simulink model "enabled_triggered_ejemplo"  (Simulink 7.1)
settings: Solver=ode45  StartTime=0.0  StopTime=10.0  RelTol=1e-3
settings Model: Creator=Usuario  LastModifiedBy=Usuario

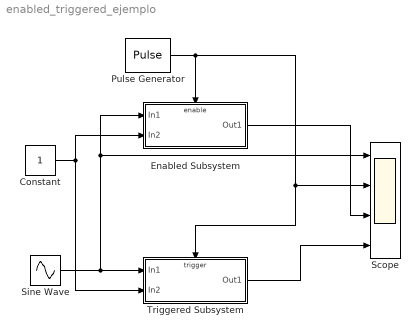
== system enabled_triggered_ejemplo ==
  Constant : Constant  OutDataType=sfix(16)  OutScaling=2^0
  Enabled Subsystem : Subsystem  TreatAsAtomicUnit=on
  Pulse Generator : DiscretePulseGenerator  PulseType=Time based  PulseWidth=50
  Scope : Scope  NumInputPorts=4
      settings: YMin=-5~-5~-5~-5  YMax=5~5~5~5
  Sine Wave : Sin  SampleTime=0
  Triggered Subsystem : Subsystem  TreatAsAtomicUnit=on
  wires:
  Sine Wave/1 -> Triggered Subsystem/1(In1), Enabled Subsystem/1(In1), Scope/1
  Pulse Generator/1 -> Enabled Subsystem/Enable, Scope/2, Triggered Subsystem/Trigger
  Constant/1 -> Enabled Subsystem/2(In2), Triggered Subsystem/2(In2)
  Enabled Subsystem/1(Out1) -> Scope/3
  Triggered Subsystem/1(Out1) -> Scope/4

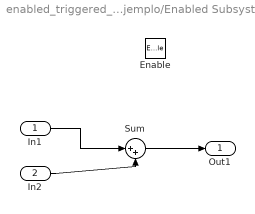
== system enabled_triggered_ejemplo/Enabled Subsystem ==
  In1 : Inport  OutDataType=sfix(16)  OutScaling=2^0
  In2 : Inport  Port=2  OutDataType=sfix(16)  OutScaling=2^0
  Enable : EnablePort
  Sum : Sum  Inputs=|++  OutDataType=sfix(16)  OutScaling=2^0
  Out1 : Outport  OutDataType=sfix(16)  OutScaling=2^0
  wires:
  In1/1 -> Sum/1
  In2/1 -> Sum/2
  Sum/1 -> Out1/1

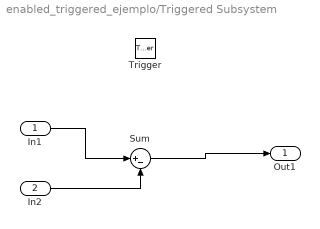
== system enabled_triggered_ejemplo/Triggered Subsystem ==
  In1 : Inport  OutDataType=sfix(16)  OutScaling=2^0
  In2 : Inport  Port=2  OutDataType=sfix(16)  OutScaling=2^0
  Trigger : TriggerPort
  Sum : Sum  Inputs=|+-  OutDataType=sfix(16)  OutScaling=2^0
  Out1 : Outport  OutDataType=sfix(16)  OutScaling=2^0
  wires:
  In1/1 -> Sum/1
  In2/1 -> Sum/2
  Sum/1 -> Out1/1
